simulink model "gerilim_bulma"  (R2018a)
settings: Solver=VariableStepAuto  StartTime=0.0  StopTime=10.0  RelTol=1e-3  AbsTol=1e-3  EnableMultiTasking=on
libraries: nesl_utility x3, fl_lib x1
settings Model: Creator=Tolga  LastModifiedBy=Tolga
settings SolverCC: AutoScaleAbsTol=off
settings DataIOCC: LimitDataPoints=on  MaxDataPoints=10000
settings OptimizationCC: LifeSpan=inf
settings DebuggingCC: AllowSymbolicDim=off  SFUnexpectedBacktrackingDiag=warning  SFNoUnconditionalDefaultTransitionDiag=warning  SFExecutionAtInitializationDiag=none
settings CodeAppCC: StateflowObjectComments=on
settings GRTTargetCC: TargetLangStandard=C89/C90 (ANSI)  GeneratePreprocessorConditionals=Disable all
settings ConfigComp: CovMetricSettings=dw  CovHtmlReporting=on  CovSaveCumulativeToWorkspaceVar=on  CovSaveSingleToWorkspaceVar=on  CovExternalEMLEnable=off  CovSFcnEnable=off
settings SimscapeCC: SimscapeLogType=all  SimscapeLogDataHistory=10000

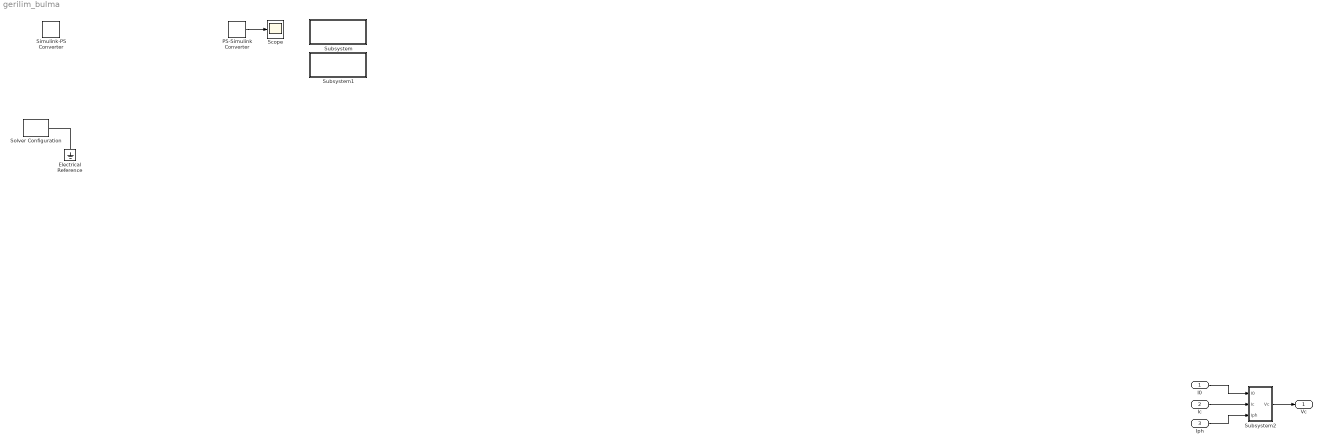
== system gerilim_bulma ==
  I0 : Inport
  Ic : Inport  Port=2
  "Iph " : Inport  Port=3
  Electrical Reference : fl_lib/Electrical/Electrical Elements/Electrical Reference
      settings: SourceProductName=Foundation Library
  PS-Simulink Converter : nesl_utility/PS-Simulink Converter  PhysicalDomain=network_engine_domain  SubClassName=ps_output  LeftPortType=input  RightPortType=output  PseudoPeriodic=off  Frequencies=[]  Unit=1  AffineConversion=off
  Scope : Scope
  Simulink-PS Converter : nesl_utility/Simulink-PS Converter  PhysicalDomain=network_engine_domain  SubClassName=ps_input  LeftPortType=input  RightPortType=output  PseudoPeriodic=off  Frequencies=[]  NoiseDistribution=none  NoiseParameters=[]  Unit=1  AffineConversion=off  FilteringAndDerivatives=zero  SimscapeFilterOrder=1  InputFilterTimeConstant=0.001  UdotUserProvided=1
  Solver Configuration : nesl_utility/Solver Configuration  PhysicalDomain=network_engine_domain  SubClassName=solver  LeftPortType=input  RightPortType=generic  Tones=[]  Harmonics=[]  SimulateNoise=off  Profile=off  UseLocalSampling=off  EnableSwitchedLinearOptims=on  FrequencyDomain=off  UseCCode=off  RelTol=0.001  AbsTol=1e-06  MinStep=1e-09  ToWorkspace=off  RevertToSquareIcSolve=off  NumHomotopyIterations=100  PhasorMode=off  PhasorModeNumHarmonics=1  DoDC=off  ResidualTolerance=1e-09  UseLocalSolver=off  LocalSolverChoice=NE_BACKWARD_EULER_ADVANCER  LocalSolverSampleTime=0.001  DoFixedCost=off  MaxNonlinIter=3  MaxModeIter=2  LinearAlgebra=Sparse  EquationFormulation=NE_TIME_EF  DelaysMemoryBudget=1024  AutomaticFiltering=on  FilteringTimeConstant=0.001
  Subsystem : Subsystem
      settings: OpenFcn=open_system('simscape')
      mask Display: disp(sprintf('Open Simscape\nLibrary'));
  Subsystem1 : Subsystem
      settings: OpenFcn=|
      | load_system('fl_lib');
      | open_system('fl_lib/Electrical');
      mask Display: disp(sprintf('Open Electrical\nLibrary'));
  Subsystem2 : Subsystem
  Vc : Outport
  wires:
  PS-Simulink Converter/1 -> Scope/1
  I0/1 -> Subsystem2/1(I0)
  Ic/1 -> Subsystem2/2(Ic)
  "Iph "/1 -> Subsystem2/3("Iph ")
  Subsystem2/1(Vc) -> Vc/1
  connections:
  Electrical Reference/LConn1 -- Solver Configuration/RConn1

== system gerilim_bulma/Subsystem ==

== system gerilim_bulma/Subsystem1 ==

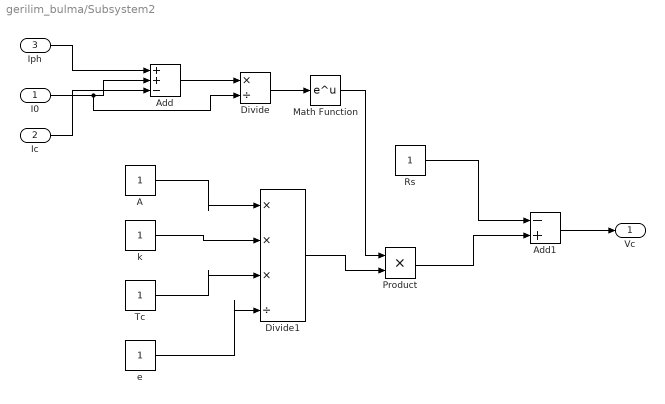
== system gerilim_bulma/Subsystem2 ==
  I0 : Inport
  Ic : Inport  Port=2
  "Iph " : Inport  Port=3
  A : Constant
  Add : Sum  Inputs=++-
  Add1 : Sum  Inputs=-+
  Divide : Product  Inputs=*/
  Divide1 : Product  Inputs=***/
  Math Function : Math  SaturateOnIntegerOverflow=on
  Product : Product
  Rs : Constant
  Tc : Constant
  e : Constant
  k : Constant
  Vc : Outport
  wires:
  Math Function/1 -> Product/1
  Ic/1 -> Add/3
  A/1 -> Divide1/1
  Rs/1 -> Add1/1
  e/1 -> Divide1/4
  I0/1 -> Divide/2, Add/2
  "Iph "/1 -> Add/1
  Add/1 -> Divide/1
  Tc/1 -> Divide1/3
  Divide1/1 -> Product/2
  Divide/1 -> Math Function/1
  k/1 -> Divide1/2
  Product/1 -> Add1/2
  Add1/1 -> Vc/1
